simulink subsystem "Dist_Vel"  (R2023b)
settings: Solver=VariableStepAuto  StartTime=0.0  StopTime=10.0  RelTol=1e-3
libraries: simulink x1
settings Model: Creator=m4ttn  LastModifiedBy=m4ttn
settings RTWCC: GPUComputeCapability=5.0

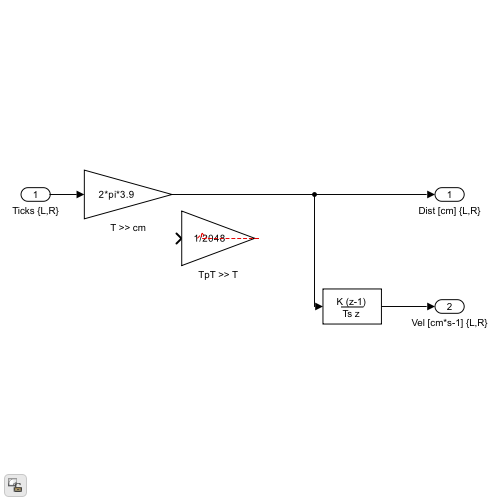
[thumbnail: Simulink's stored preview of the top-level diagram]
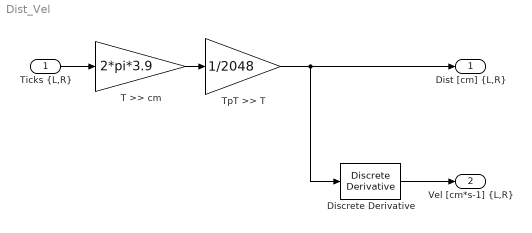
== system Dist_Vel ==
  "Ticks {L,R}" : Inport  OutDataTypeStr=int32
  Discrete Derivative : simulink/Discrete/Discrete Derivative  gainval=1.0  ICPrevScaledInput=0.0  OutMin=[]  OutMax=[]  OutDataTypeStr=int32  OutputDataTypeScalingMode=int32  OutDataType=fixdt(1, 16)  OutScaling=2^-10  DoSatur=off
  T >> cm : Gain  Gain=2*pi*3.9  OutDataTypeStr=int32
  TpT >> T : Gain  Gain=1/2048  OutDataTypeStr=int16
  "Dist [cm] {L,R}" : Outport  OutDataTypeStr=int32
  "Vel [cm*s-1] {L,R}" : Outport  Port=2  OutDataTypeStr=int32
  wires:
  "Ticks {L,R}"/1 -> T >> cm/1
  Discrete Derivative/1 -> "Vel [cm*s-1] {L,R}"/1
  T >> cm/1 -> TpT >> T/1
  TpT >> T/1 -> Discrete Derivative/1, "Dist [cm] {L,R}"/1
